simulink model "wholev5"  (R2018b)
settings: Solver=ode45  StartTime=0.0  StopTime=200  FixedStep=0.01  RelTol=1e-3
libraries: aerolibatmos2 x4
settings Model: Creator=hou2  LastModifiedBy=wq
settings DataIOCC: LimitDataPoints=on
settings OptimizationCC: DefaultParameterBehavior=Inlined  UseDivisionForNetSlopeComputation=on  UseFloatMulNetSlope=on  InlineInvariantSignals=on  PassReuseOutputArgsAs=Individual arguments  ZeroExternalMemoryAtStartup=off  ZeroInternalMemoryAtStartup=off  NoFixptDivByZeroProtection=on  EfficientFloat2IntCast=on  LifeSpan=1  OptimizeBlockOrder=speed  DifferentSizesBufferReuse=on
settings DebuggingCC: ParameterTunabilityLossMsg=error  AllowSymbolicDim=off  SFUnexpectedBacktrackingDiag=warning  SFNoUnconditionalDefaultTransitionDiag=warning  SFExecutionAtInitializationDiag=none
settings HardwareCC: ProdBitPerLong=64  ProdLongLongMode=on  ProdHWDeviceType=Intel->x86-64 (Linux 64)
settings ModelReferenceCC: PropagateSignalLabelsOutOfModel=off
settings SFSimCC: SimUseLocalCustomCode=off  MATLABDynamicMemAlloc=off
settings RTWCC: SystemTargetFile=ert.tlc  GenCodeOnly=on  TemplateMakefile=ert_default_tmf  GenerateReport=on  RTWUseLocalCustomCode=off  BuildConfiguration=Faster Runs  IncludeHyperlinkInReport=on  LaunchReport=on  TargetLang=C++  GenerateTraceInfo=on  GenerateTraceReport=on  GenerateTraceReportSl=on  GenerateTraceReportSf=on  GenerateTraceReportEml=on
settings CodeAppCC: ForceParamTrailComments=on  IgnoreCustomStorageClasses=off  OperatorAnnotations=on  SimulinkDataObjDesc=on  SFDataObjDesc=on  CustomSymbolStrGlobalVar=rt$N$M  CustomSymbolStrType=$N$M  CustomSymbolStrFcn=$N$M$F  CustomSymbolStrMacro=$N$M  InsertBlockDesc=on
settings ERTTargetCC: TargetLangStandard=C++03 (ISO)  GenerateSampleERTMain=on  IncludeMdlTerminateFcn=off  CombineSignalStateStructs=on  MultiInstanceERTCode=on  CodeInterfacePackaging=C++ class  SupportComplex=off  SupportContinuousTime=on  SupportNonInlinedSFcns=on  InlinedParameterPlacement=NonHierarchical  RootIOFormat=Structure reference  RTWCAPISignals=on  RTWCAPIParams=on  RTWCAPIStates=on  RTWCAPIRootIO=on  ERTCustomFileTemplate=example_file_process.tlc  ERTFilePackagingFormat=CompactWithDataFile
settings ConfigComp: CovMetricSettings=dw  CovHtmlReporting=on  CovSaveCumulativeToWorkspaceVar=on  CovSaveSingleToWorkspaceVar=on  CovExternalEMLEnable=off

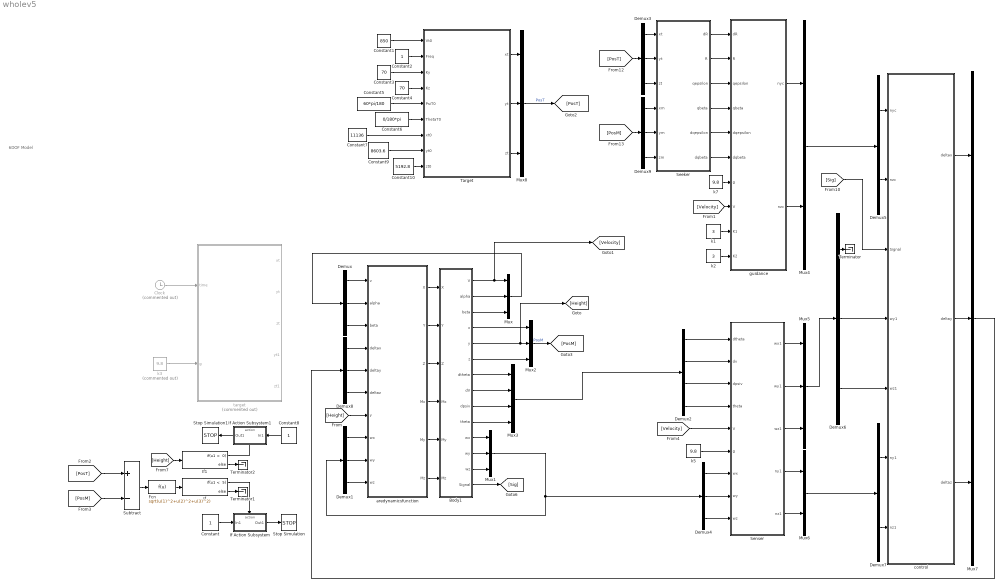
== system wholev5 ==
  note: 6DOF Model
  Body1 : Subsystem
  Clock : Clock  Commented=on
  Constant : Constant
  Constant1 : Constant  Value=850
  Constant10 : Constant  Value=5192.8
  Constant2 : Constant
  Constant3 : Constant  Value=70
  Constant4 : Constant  Value=70
  Constant5 : Constant  Value=60*pi/180
  Constant6 : Constant  Value=0/180*pi
  Constant7 : Constant  Value=11136
  Constant8 : Constant
  Constant9 : Constant  Value=8603.6
  Demux{,1,3..4,6,8..9} (7 alike) : Demux  Outputs=3
  Demux2 : Demux
  Demux5 : Demux  Outputs=2
  Demux7 : Demux  Outputs=2
  Fcn : Fcn  Expr=sqrt(u(1)^2+u(2)^2+u(3)^2)
  If : If  IfExpression="u1 <  5"
  If Action Subsystem : Subsystem  TreatAsAtomicUnit=on
  If Action Subsystem1 : Subsystem  TreatAsAtomicUnit=on
  If1 : If  IfExpression="u1 <  0"
  Mux{,1..2,5,7..8} (6 alike) : Mux  Inputs=3
  Mux3 : Mux
  Mux4 : Mux  Inputs=2
  Mux6 : Mux  Inputs=2
  Seeker : Subsystem
  Senser : Subsystem
  Stop Simulation : Stop
  Stop Simulation1 : Stop
  Subtract : Sum  Inputs=+-
  Target : Subsystem
  Terminator : Terminator
  Terminator1 : Terminator
  Terminator2 : Terminator
  aredynamicsfunction : Subsystem
  control : Subsystem
  guidance : Subsystem
  k1 : Constant  Value=3
  k2 : Constant  Value=3
  k3 : Constant  Commented=on  Value=9.8
  k5 : Constant  Value=9.8
  k7 : Constant  Value=9.8
  target : Subsystem  Commented=on
  wires:
  aredynamicsfunction/6(Mz) -> Body1/6(Mz)
  aredynamicsfunction/5(My) -> Body1/5(My)
  aredynamicsfunction/4(Mx) -> Body1/4(Mx)
  aredynamicsfunction/3(Z) -> Body1/3(Z)
  aredynamicsfunction/1(X) -> Body1/1(X)
  aredynamicsfunction/2(Y) -> Body1/2(Y)
  Seeker/3(qepsilon) -> guidance/3(qepsilon)
  Seeker/2(R) -> guidance/2(R)
  Seeker/6(dqbeta) -> guidance/6(dqbeta)
  Seeker/1(dR) -> guidance/1(dR)
  Seeker/4(qbeta) -> guidance/4(qbeta)
  Seeker/5(dqepsilon) -> guidance/5(dqepsilon)
  k1/1 -> guidance/9(K1)
  [Velocity] -> guidance/8(V)
  k2/1 -> guidance/10(K2)
  k7/1 -> guidance/7(g)
  Body1/1(V) -> Mux/1, [Velocity]
  Body1/2(alpha) -> Mux/2
  Body1/3(beta) -> Mux/3
  Mux/1 -> Demux/1
  Body1/11(wx) -> Mux1/1
  Body1/12(wy) -> Mux1/2
  Body1/13(wz) -> Mux1/3
  Mux1/1 -> Demux1/1, Demux4/1
  Body1/4(x) -> Mux2/1
  Body1/5(y) -> [Height], Mux2/2
  Body1/6(z) -> Mux2/3
  Mux2/1 -> [PosM]  "PosM"
  Body1/7(dtheta) -> Mux3/1
  Body1/8(dV) -> Mux3/2
  Body1/9(dpsiv) -> Mux3/3
  Body1/10(theta) -> Mux3/4
  [PosT] -> Subtract/1
  [PosM] -> Subtract/2
  Subtract/1 -> Fcn/1
  Fcn/1 -> If/1
  If/1 -> If Action Subsystem/Action
  If Action Subsystem/1(Out1) -> Stop Simulation/1
  If/2 -> Terminator1/1
  Constant/1 -> If Action Subsystem/1(In1)
  Demux2/1 -> Senser/1(dtheta)
  Demux2/2 -> Senser/2(dv)
  Demux2/3 -> Senser/3(dpsiv)
  Demux2/4 -> Senser/4(theta)
  [Velocity] -> Senser/5(V)
  k5/1 -> Senser/6(g)
  Demux4/1 -> Senser/7(wx)
  Demux4/2 -> Senser/8(wy)
  Demux4/3 -> Senser/9(wz)
  guidance/1(nyc) -> Mux4/1
  guidance/2(nzc) -> Mux4/2
  Senser/2(wy1) -> Mux5/2
  Senser/3(wz1) -> Mux5/3
  Senser/1("wx1 ") -> Mux5/1
  Senser/4(ny1) -> Mux6/1
  Senser/5(nz1) -> Mux6/2
  control/3(deltaz) -> Mux7/3
  control/2(deltay) -> Mux7/2
  control/1(deltax) -> Mux7/1
  Mux7/1 -> Demux8/1
  Demux/1 -> aredynamicsfunction/1(v)
  Demux/2 -> aredynamicsfunction/2(alpha)
  Demux/3 -> aredynamicsfunction/3(beta)
  Demux8/1 -> aredynamicsfunction/4(deltax)
  Demux8/2 -> aredynamicsfunction/5(deltay)
  Demux8/3 -> aredynamicsfunction/6(deltaz)
  Demux1/1 -> aredynamicsfunction/8(wx)
  Demux1/2 -> aredynamicsfunction/9(wy)
  Demux1/3 -> aredynamicsfunction/10(wz)
  [Height] -> aredynamicsfunction/7(y)
  Demux5/1 -> control/1(nyc)
  Demux5/2 -> control/2(nzc)
  Mux4/1 -> Demux5/1
  Demux6/2 -> control/4(wy1)
  Demux6/3 -> control/5(wz1)
  Mux5/1 -> Demux6/1
  Demux7/1 -> control/6(ny1)
  Demux7/2 -> control/7(nz1)
  Mux6/1 -> Demux7/1
  Constant1/1 -> Target/1(Vt0)
  Constant2/1 -> Target/2(Freq)
  Constant3/1 -> Target/3(Ky)
  Constant4/1 -> Target/4(Kz)
  Constant5/1 -> Target/5(PsiT0)
  Constant6/1 -> Target/6(ThetaT0)
  Clock/1 -> target/1(time)
  k3/1 -> target/2(g)
  Mux8/1 -> [PosT]  "PosT"
  [Height] -> If1/1
  If1/2 -> Terminator2/1
  If1/1 -> If Action Subsystem1/Action
  Constant8/1 -> If Action Subsystem1/1(In1)
  If Action Subsystem1/1(Out1) -> Stop Simulation1/1
  Target/1(xt) -> Mux8/1
  Target/2(yt) -> Mux8/2
  Target/3(zt) -> Mux8/3
  Mux3/1 -> Demux2/1
  Constant7/1 -> Target/7(xt0)
  Constant9/1 -> Target/8(yt0)
  Constant10/1 -> Target/9(zt0)
  Demux6/1 -> Terminator/1
  Body1/14(Signal) -> [Sig]
  [Sig] -> control/3(Signal)
  Demux3/1 -> Seeker/1(xt)
  Demux3/2 -> Seeker/2(yt)
  Demux3/3 -> Seeker/3(zt)
  Demux9/1 -> Seeker/4(xm)
  Demux9/3 -> Seeker/6(zm)
  Demux9/2 -> Seeker/5(ym)
  [PosT] -> Demux3/1
  [PosM] -> Demux9/1

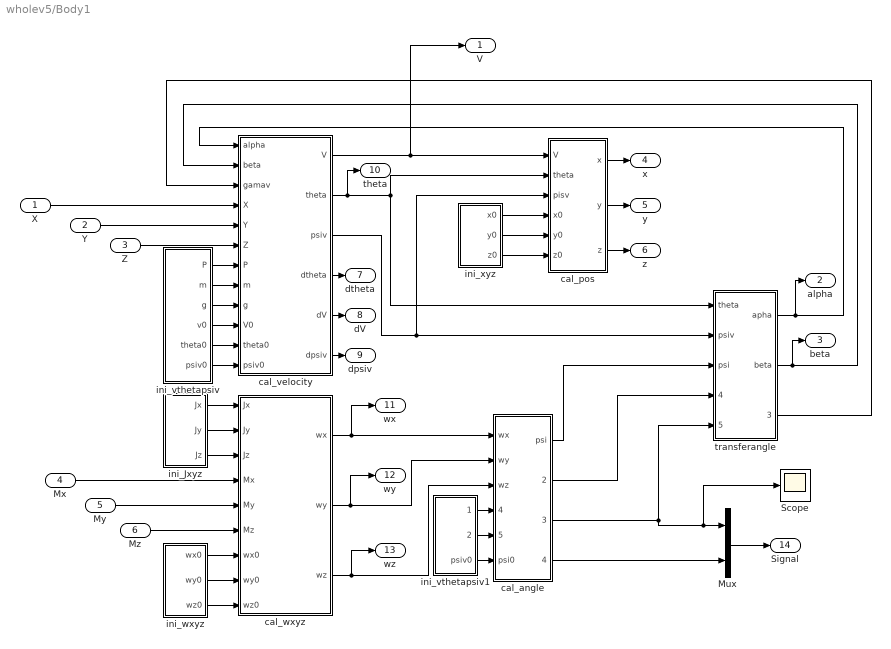
== system wholev5/Body1 ==
  X : Inport
  Y : Inport  Port=2
  Z : Inport  Port=3
  Mx : Inport  Port=4
  My : Inport  Port=5
  Mz : Inport  Port=6
  Mux : Mux  Inputs=2
  Scope : Scope
  cal_angle : Subsystem
  cal_pos : Subsystem
  cal_velocity : Subsystem
  cal_wxyz : Subsystem
  ini_Jxyz : Subsystem
  ini_vthetapsiv : Subsystem
  ini_vthetapsiv1 : Subsystem
  ini_wxyz : Subsystem
  ini_xyz : Subsystem
  transferangle : Subsystem
  V : Outport
  alpha : Outport  Port=2
  beta : Outport  Port=3
  x : Outport  Port=4
  y : Outport  Port=5
  z : Outport  Port=6
  dtheta : Outport  Port=7
  dV : Outport  Port=8
  dpsiv : Outport  Port=9
  theta : Outport  Port=10
  wx : Outport  Port=11
  wy : Outport  Port=12
  wz : Outport  Port=13
  Signal : Outport  Port=14
  wires:
  transferangle/3(gamav) -> cal_velocity/3(gamav)
  cal_velocity/2(theta) -> theta/1, transferangle/1(theta), cal_pos/2(theta)
  cal_velocity/3(psiv) -> cal_pos/3(pisv), transferangle/2(psiv)
  cal_velocity/1(V) -> cal_pos/1(V), V/1
  cal_wxyz/1(wx) -> cal_angle/1(wx), wx/1
  cal_wxyz/2(wy) -> cal_angle/2(wy), wy/1
  cal_wxyz/3(wz) -> cal_angle/3(wz), wz/1
  cal_angle/3(gama) -> Scope/1, Mux/1, transferangle/5(gama)
  cal_angle/2(Ctheta) -> transferangle/4(Ctheta)
  cal_angle/1(psi) -> transferangle/3(psi)
  transferangle/2(beta) -> beta/1, cal_velocity/2(beta)
  transferangle/1(apha) -> alpha/1, cal_velocity/1(alpha)
  cal_pos/1(x) -> x/1
  Y/1 -> cal_velocity/5(Y)
  Mx/1 -> cal_wxyz/4(Mx)
  Mz/1 -> cal_wxyz/6(Mz)
  Z/1 -> cal_velocity/6(Z)
  My/1 -> cal_wxyz/5(My)
  X/1 -> cal_velocity/4(X)
  ini_Jxyz/3(Jz) -> cal_wxyz/3(Jz)
  ini_Jxyz/2(Jy) -> cal_wxyz/2(Jy)
  ini_Jxyz/1(Jx) -> cal_wxyz/1(Jx)
  ini_vthetapsiv1/1(gama0) -> cal_angle/4(gama0)
  ini_wxyz/2(wy0) -> cal_wxyz/8(wy0)
  ini_wxyz/3(wz0) -> cal_wxyz/9(wz0)
  ini_wxyz/1(wx0) -> cal_wxyz/7(wx0)
  ini_xyz/1(x0) -> cal_pos/4(x0)
  ini_xyz/3(z0) -> cal_pos/6(z0)
  ini_xyz/2(y0) -> cal_pos/5(y0)
  cal_pos/2(y) -> y/1
  ini_vthetapsiv1/3(psiv0) -> cal_angle/6(psi0)
  ini_vthetapsiv1/2(Ctheta0) -> cal_angle/5(pha0)
  cal_pos/3(z) -> z/1
  cal_velocity/4(dtheta) -> dtheta/1
  cal_velocity/5(dV) -> dV/1
  cal_velocity/6(dpsiv) -> dpsiv/1
  ini_vthetapsiv/1(P) -> cal_velocity/7(P)
  ini_vthetapsiv/2(m) -> cal_velocity/8(m)
  ini_vthetapsiv/3(g) -> cal_velocity/9(g)
  ini_vthetapsiv/4(v0) -> cal_velocity/10(V0)
  ini_vthetapsiv/5(theta0) -> cal_velocity/11(theta0)
  ini_vthetapsiv/6(psiv0) -> cal_velocity/12(psiv0)
  cal_angle/4(Dgama) -> Mux/2
  Mux/1 -> Signal/1

== system wholev5/If Action Subsystem ==
  In1 : Inport
  Action Port : ActionPort  ActionType=then
  Out1 : Outport
  wires:
  In1/1 -> Out1/1

== system wholev5/If Action Subsystem1 ==
  In1 : Inport
  Action Port : ActionPort  ActionType=then
  Out1 : Outport
  wires:
  In1/1 -> Out1/1

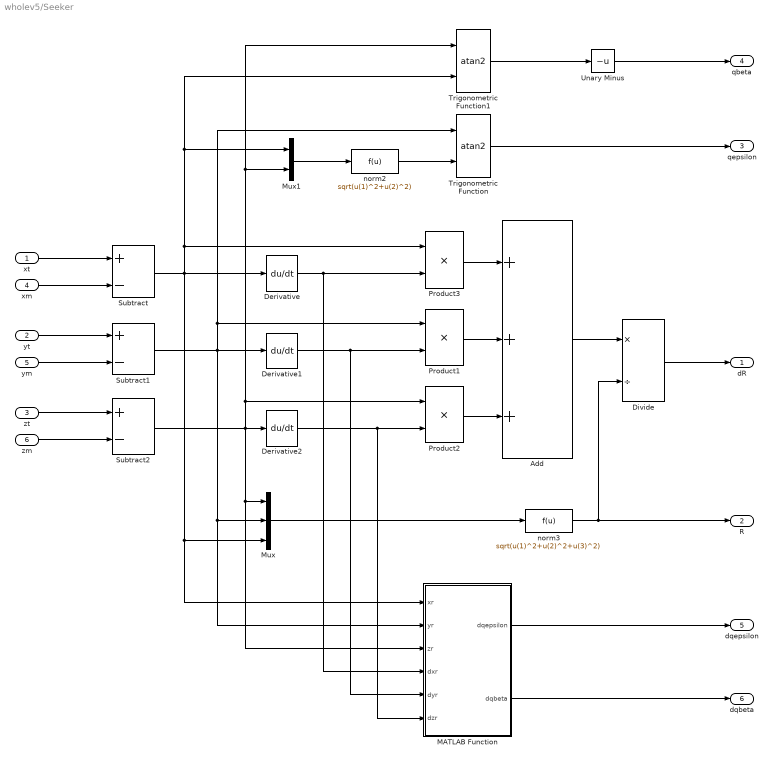
== system wholev5/Seeker ==
  xt : Inport
  yt : Inport  Port=2
  zt : Inport  Port=3
  xm : Inport  Port=4
  ym : Inport  Port=5
  zm : Inport  Port=6
  Add : Sum  Inputs=3
  Derivative : Derivative
  Derivative1 : Derivative
  Derivative2 : Derivative
  Divide : Product  Inputs=*/
  MATLAB Function : MATLAB Function  TreatAsAtomicUnit=on
  Mux : Mux  Inputs=3
  Mux1 : Mux  Inputs=2
  Product1 : Product
  Product2 : Product
  Product3 : Product
  Subtract : Sum  Inputs=+-
  Subtract1 : Sum  Inputs=+-
  Subtract2 : Sum  Inputs=+-
  Trigonometric Function : Trigonometry  Operator=atan2
  Trigonometric Function1 : Trigonometry  Operator=atan2
  Unary Minus : UnaryMinus
  norm2 : Fcn  Expr=sqrt(u(1)^2+u(2)^2)
  norm3 : Fcn  Expr=sqrt(u(1)^2+u(2)^2+u(3)^2)
  dR : Outport
  R : Outport  Port=2
  qepsilon : Outport  Port=3
  qbeta : Outport  Port=4
  dqepsilon : Outport  Port=5
  dqbeta : Outport  Port=6
  wires:
  Trigonometric Function/1 -> qepsilon/1
  Trigonometric Function1/1 -> Unary Minus/1
  Mux1/1 -> norm2/1
  Derivative/1 -> MATLAB Function/4(dxr), Product3/2
  Mux/1 -> norm3/1
  xm/1 -> Subtract/2
  Product3/1 -> Add/1
  zt/1 -> Subtract2/1
  Subtract1/1 -> MATLAB Function/2(yr), Mux/2, Derivative1/1, Trigonometric Function/1, Product1/1
  Subtract2/1 -> MATLAB Function/3(zr), Mux/1, Trigonometric Function1/1, Mux1/2, Product2/1, Derivative2/1
  Product1/1 -> Add/2
  Product2/1 -> Add/3
  Unary Minus/1 -> qbeta/1
  Divide/1 -> dR/1
  Add/1 -> Divide/1
  xt/1 -> Subtract/1
  ym/1 -> Subtract1/2
  Subtract/1 -> Mux/3, MATLAB Function/1(xr), Derivative/1, Trigonometric Function1/2, Mux1/1, Product3/1
  zm/1 -> Subtract2/2
  Derivative1/1 -> MATLAB Function/5(dyr), Product1/2
  yt/1 -> Subtract1/1
  norm2/1 -> Trigonometric Function/2
  norm3/1 -> R/1, Divide/2
  Derivative2/1 -> MATLAB Function/6(dzr), Product2/2
  MATLAB Function/2(dqbeta) -> dqbeta/1
  MATLAB Function/1(dqepsilon) -> dqepsilon/1

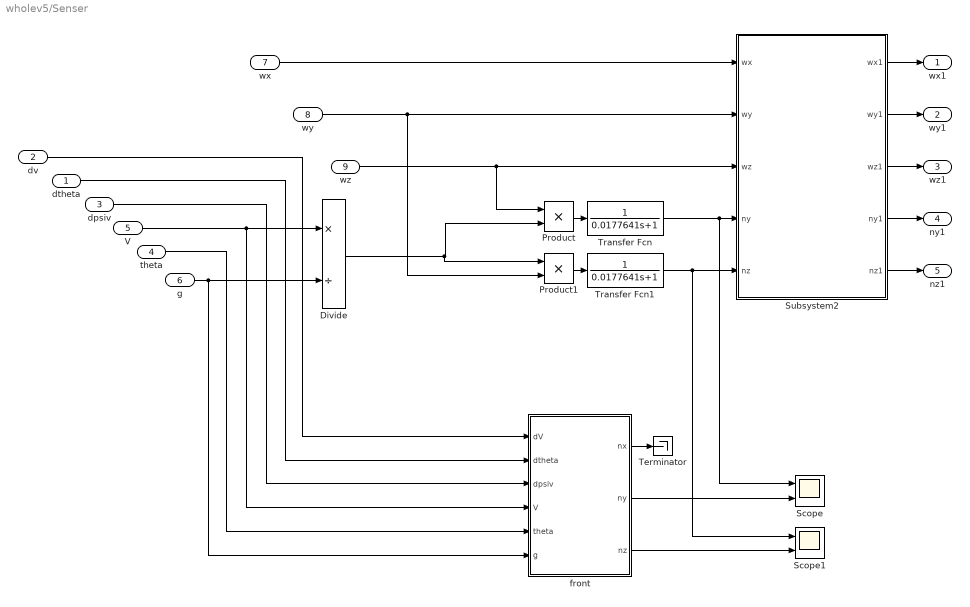
== system wholev5/Senser ==
  dtheta : Inport
  dv : Inport  Port=2
  dpsiv : Inport  Port=3
  theta : Inport  Port=4
  V : Inport  Port=5
  g : Inport  Port=6
  wx : Inport  Port=7
  wy : Inport  Port=8
  wz : Inport  Port=9
  Divide : Product  Inputs=*/
  Product : Product
  Product1 : Product
  Scope : Scope  NumInputPorts=2
  Scope1 : Scope  NumInputPorts=2
  Subsystem2 : Subsystem
  Terminator : Terminator
  Transfer Fcn : TransferFcn  Denominator=[0.0177641 1]
  Transfer Fcn1 : TransferFcn  Denominator=[0.0177641 1]
  front : Subsystem
  "wx1 " : Outport
  wy1 : Outport  Port=2
  wz1 : Outport  Port=3
  ny1 : Outport  Port=4
  nz1 : Outport  Port=5
  wires:
  wz/1 -> Product/1, Subsystem2/3(wz)
  dtheta/1 -> front/2(dtheta)
  wx/1 -> Subsystem2/1(wx)
  wy/1 -> Product1/2, Subsystem2/2(wy)
  dpsiv/1 -> front/3(dpsiv)
  theta/1 -> front/5(theta)
  dv/1 -> front/1(dV)
  Subsystem2/2(wy1) -> wy1/1
  V/1 -> front/4(V), Divide/1
  Subsystem2/1(wx1) -> "wx1 "/1
  Subsystem2/5(nz1) -> nz1/1
  g/1 -> front/6(g), Divide/2
  Subsystem2/3(wz1) -> wz1/1
  front/2(ny) -> Scope/2
  front/3(nz) -> Scope1/2
  Subsystem2/4(ny1) -> ny1/1
  front/1(nx) -> Terminator/1
  Transfer Fcn/1 -> Scope/1, Subsystem2/4(ny)
  Transfer Fcn1/1 -> Scope1/1, Subsystem2/5(nz)
  Product/1 -> Transfer Fcn/1
  Product1/1 -> Transfer Fcn1/1
  Divide/1 -> Product1/1, Product/2

== system wholev5/Target ==
  Vt0 : Inport
  Freq : Inport  Port=2
  Ky : Inport  Port=3
  Kz : Inport  Port=4
  PsiT0 : Inport  Port=5
  ThetaT0 : Inport  Port=6
  xt0 : Inport  Port=7
  yt0 : Inport  Port=8
  zt0 : Inport  Port=9
  Clock : Clock
  Integrator{,1..5} (6 alike) : Integrator  InitialConditionSource=external
  MATLAB Function : MATLAB Function  TreatAsAtomicUnit=on
  xt : Outport
  yt : Outport  Port=2
  zt : Outport  Port=3
  wires:
  zt0/1 -> Integrator2/2
  MATLAB Function/4(dx) -> Integrator4/1
  yt0/1 -> Integrator3/2
  Clock/1 -> MATLAB Function/4(t)
  Integrator1/1 -> MATLAB Function/3(Psi)
  MATLAB Function/2(dTheta) -> Integrator/1
  ThetaT0/1 -> Integrator/2
  PsiT0/1 -> Integrator1/2
  Freq/1 -> MATLAB Function/5(w)
  xt0/1 -> Integrator4/2
  Integrator3/1 -> yt/1
  Integrator4/1 -> xt/1
  Integrator/1 -> MATLAB Function/2(Theta)
  Kz/1 -> MATLAB Function/7(Kz)
  MATLAB Function/6(dz) -> Integrator2/1
  Integrator2/1 -> zt/1
  Ky/1 -> MATLAB Function/6(Ky)
  MATLAB Function/5(dy) -> Integrator3/1
  MATLAB Function/3(dPsi) -> Integrator1/1
  Vt0/1 -> Integrator5/2
  MATLAB Function/1(dV) -> Integrator5/1
  Integrator5/1 -> MATLAB Function/1(V)

== system wholev5/aredynamicsfunction ==
  v : Inport
  alpha : Inport  Port=2
  beta : Inport  Port=3
  deltax : Inport  Port=4
  deltay : Inport  Port=5
  deltaz : Inport  Port=6
  y : Inport  Port=7
  wx : Inport  Port=8
  wy : Inport  Port=9
  wz : Inport  Port=10
  Constant : Constant  Value=0
  cal_forceXYZ : Subsystem
  cal_momentMXZY : Subsystem
  X : Outport
  Y : Outport  Port=2
  Z : Outport  Port=3
  Mx : Outport  Port=4
  My : Outport  Port=5
  Mz : Outport  Port=6
  wires:
  Constant/1 -> cal_forceXYZ/3(Cx)
  v/1 -> cal_momentMXZY/2(V), cal_forceXYZ/2(V)
  cal_momentMXZY/1(Mx) -> Mx/1
  cal_forceXYZ/1(X) -> X/1
  cal_forceXYZ/2(Y) -> Y/1
  cal_momentMXZY/2(My) -> My/1
  cal_momentMXZY/3(Mz) -> Mz/1
  wz/1 -> cal_momentMXZY/10(wz)
  wx/1 -> cal_momentMXZY/8(wx)
  cal_forceXYZ/3(Z) -> Z/1
  deltaz/1 -> cal_momentMXZY/7(deltaz), cal_forceXYZ/7(deltaz)
  beta/1 -> cal_forceXYZ/5(beta), cal_momentMXZY/4(beta)
  deltay/1 -> cal_momentMXZY/6(deltay), cal_forceXYZ/6(deltay)
  alpha/1 -> cal_momentMXZY/3(alpha), cal_forceXYZ/4(alpha)
  y/1 -> cal_forceXYZ/1(y), cal_momentMXZY/1(y)
  wy/1 -> cal_momentMXZY/9(wy)
  deltax/1 -> cal_momentMXZY/5(deltax)

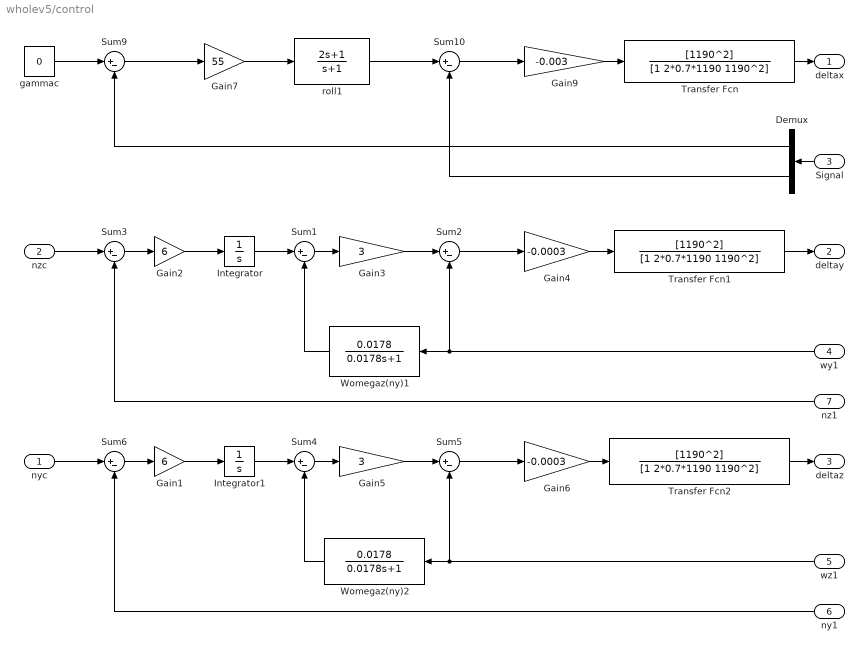
== system wholev5/control ==
  nyc : Inport
  nzc : Inport  Port=2
  Signal : Inport  Port=3
  wy1 : Inport  Port=4
  wz1 : Inport  Port=5
  ny1 : Inport  Port=6
  nz1 : Inport  Port=7
  " Womegaz(ny)1" : TransferFcn  Numerator=[0.0178]  Denominator=[0.0178 1]
  " Womegaz(ny)2" : TransferFcn  Numerator=[0.0178]  Denominator=[0.0178 1]
  Demux : Demux  Outputs=2
  Gain1 : Gain  Gain=6
  Gain2 : Gain  Gain=6
  Gain3 : Gain  Gain=3
  Gain4 : Gain  Gain=-0.0003
  Gain5 : Gain  Gain=3
  Gain6 : Gain  Gain=-0.0003
  Gain7 : Gain  Gain=55
  Gain9 : Gain  Gain=-0.003
  Integrator : Integrator
  Integrator1 : Integrator
  Sum{1..6,9..10} (8 alike) : Sum  Inputs=|+-
  Transfer Fcn : TransferFcn  Numerator=[1190^2]  Denominator=[1 2*0.7*1190 1190^2]
  Transfer Fcn1 : TransferFcn  Numerator=[1190^2]  Denominator=[1 2*0.7*1190 1190^2]
  Transfer Fcn2 : TransferFcn  Numerator=[1190^2]  Denominator=[1 2*0.7*1190 1190^2]
  gammac : Constant  Value=0
  roll1 : TransferFcn  Numerator=[2 1]  Denominator=[1 1]
  deltax : Outport
  deltay : Outport  Port=2
  deltaz : Outport  Port=3
  wires:
  Transfer Fcn/1 -> deltax/1
  Transfer Fcn1/1 -> deltay/1
  Transfer Fcn2/1 -> deltaz/1
  Gain2/1 -> Integrator/1
  Integrator/1 -> Sum1/1
  Sum2/1 -> Gain4/1
  Gain3/1 -> Sum2/1
  Sum1/1 -> Gain3/1
  Sum3/1 -> Gain2/1
  nzc/1 -> Sum3/1
  nz1/1 -> Sum3/2
  " Womegaz(ny)1"/1 -> Sum1/2
  wy1/1 -> Sum2/2, " Womegaz(ny)1"/1
  Gain4/1 -> Transfer Fcn1/1
  Gain1/1 -> Integrator1/1
  Integrator1/1 -> Sum4/1
  Sum5/1 -> Gain6/1
  Gain5/1 -> Sum5/1
  Sum4/1 -> Gain5/1
  Sum6/1 -> Gain1/1
  nyc/1 -> Sum6/1
  ny1/1 -> Sum6/2
  " Womegaz(ny)2"/1 -> Sum4/2
  wz1/1 -> Sum5/2, " Womegaz(ny)2"/1
  Gain6/1 -> Transfer Fcn2/1
  Signal/1 -> Demux/1
  Gain7/1 -> roll1/1
  Demux/1 -> Sum9/2
  roll1/1 -> Sum10/1
  Sum9/1 -> Gain7/1
  Sum10/1 -> Gain9/1
  gammac/1 -> Sum9/1
  Demux/2 -> Sum10/2
  Gain9/1 -> Transfer Fcn/1

== system wholev5/guidance ==
  dR : Inport
  R : Inport  Port=2
  qepsilon : Inport  Port=3
  qbeta : Inport  Port=4
  dqepsilon : Inport  Port=5
  dqbeta : Inport  Port=6
  g : Inport  Port=7
  V : Inport  Port=8
  K1 : Inport  Port=9
  K2 : Inport  Port=10
  Divide : Product  Inputs=/*
  Product : Product  Inputs=3
  Product1 : Product  Inputs=3
  Terminator{,1..3} (4 alike) : Terminator
  nyc : Outport
  nzc : Outport  Port=2
  wires:
  R/1 -> Terminator1/1
  qepsilon/1 -> Terminator2/1
  g/1 -> Divide/1
  dR/1 -> Terminator/1
  V/1 -> Divide/2
  qbeta/1 -> Terminator3/1
  Product1/1 -> nzc/1
  dqbeta/1 -> Product1/3
  dqepsilon/1 -> Product/1
  K2/1 -> Product1/2
  K1/1 -> Product/2
  Divide/1 -> Product1/1, Product/3
  Product/1 -> nyc/1

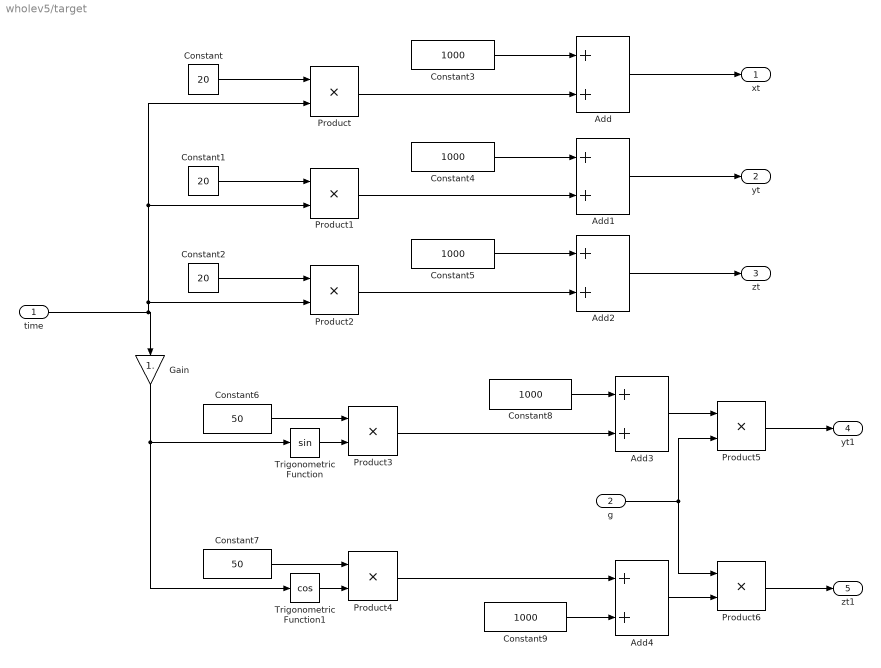
== system wholev5/target ==
  time : Inport
  g : Inport  Port=2
  Add{,1..4} (5 alike) : Sum
  Constant : Constant  Value=20
  Constant1 : Constant  Value=20
  Constant2 : Constant  Value=20
  Constant{3..5,8..9} (5 alike) : Constant  Value=1000
  Constant6 : Constant  Value=50
  Constant7 : Constant  Value=50
  Gain : Gain  Gain=1.
  Product{,1..6} (7 alike) : Product
  Trigonometric Function : Trigonometry
  Trigonometric Function1 : Trigonometry  Operator=cos
  xt : Outport
  yt : Outport  Port=2
  zt : Outport  Port=3
  yt1 : Outport  Port=4
  zt1 : Outport  Port=5
  wires:
  Product6/1 -> zt1/1
  Trigonometric Function/1 -> Product3/2
  Constant7/1 -> Product4/1
  Constant3/1 -> Add/1
  Constant5/1 -> Add2/1
  Constant/1 -> Product/1
  Product2/1 -> Add2/2
  Constant4/1 -> Add1/1
  Product1/1 -> Add1/2
  g/1 -> Product6/1, Product5/2
  Trigonometric Function1/1 -> Product4/2
  Constant6/1 -> Product3/1
  Add2/1 -> zt/1
  Constant1/1 -> Product1/1
  Product5/1 -> yt1/1
  Product/1 -> Add/2
  Constant2/1 -> Product2/1
  Add1/1 -> yt/1
  time/1 -> Gain/1, Product/2, Product1/2, Product2/2
  Add/1 -> xt/1
  Gain/1 -> Trigonometric Function/1, Trigonometric Function1/1
  Constant8/1 -> Add3/1
  Product3/1 -> Add3/2
  Add3/1 -> Product5/1
  Constant9/1 -> Add4/2
  Product4/1 -> Add4/1
  Add4/1 -> Product6/2

== system wholev5/Body1/cal_angle ==
  wx : Inport
  wy : Inport  Port=2
  wz : Inport  Port=3
  gama0 : Inport  Port=4
  pha0 : Inport  Port=5
  psi0 : Inport  Port=6
  Divide : Product  Inputs=**
  Divide1 : Product  Inputs=**
  Divide2 : Product  Inputs=/*
  Integrator : Integrator  InitialConditionSource=external
  Subtract : Sum  Inputs=+-
  Trigonometric Function : Trigonometry  Operator=cos
  Trigonometric Function1 : Trigonometry
  Trigonometric Function2 : Trigonometry  Operator=cos
  cal_Ctheta : Subsystem
  psi : Outport
  Ctheta : Outport  Port=2
  gama : Outport  Port=3
  Dgama : Outport  Port=4
  wires:
  Trigonometric Function/1 -> Divide/1
  wy/1 -> cal_Ctheta/2(wy), Divide/2
  wz/1 -> cal_Ctheta/4(wz), Divide1/2
  cal_Ctheta/2(gama) -> Trigonometric Function1/1, Trigonometric Function/1, gama/1
  Divide/1 -> Subtract/1
  psi0/1 -> Integrator/2
  Integrator/1 -> psi/1
  Trigonometric Function1/1 -> Divide1/1
  Trigonometric Function2/1 -> Divide2/1
  wx/1 -> cal_Ctheta/1(wx)
  Subtract/1 -> Divide2/2
  Divide1/1 -> Subtract/2
  cal_Ctheta/1(Ctheta) -> Trigonometric Function2/1, Ctheta/1
  pha0/1 -> cal_Ctheta/5(pha0)
  Divide2/1 -> Integrator/1
  gama0/1 -> cal_Ctheta/3(gama0)
  cal_Ctheta/3(Dgama) -> Dgama/1

== system wholev5/Body1/cal_pos ==
  note: x坐标的初始值
  note: z坐标的初始值
  V : Inport
  theta : Inport  Port=2
  pisv : Inport  Port=3
  x0 : Inport  Port=4
  y0 : Inport  Port=5
  z0 : Inport  Port=6
  Gain2 : Gain  Gain=-1
  Integrator : Integrator  InitialConditionSource=external
  Integrator1 : Integrator  InitialConditionSource=external
  Integrator2 : Integrator  InitialConditionSource=external
  Product : Product  Inputs=3
  Product1 : Product
  Product2 : Product  Inputs=3
  Trigonometric Function : Trigonometry  Operator=cos
  Trigonometric Function1 : Trigonometry  Operator=cos
  Trigonometric Function2 : Trigonometry
  Trigonometric Function3 : Trigonometry
  x : Outport
  y : Outport  Port=2
  z : Outport  Port=3
  wires:
  Integrator/1 -> x/1
  theta/1 -> Trigonometric Function2/1, Trigonometric Function/1
  pisv/1 -> Trigonometric Function3/1, Trigonometric Function1/1
  Trigonometric Function1/1 -> Product/2
  Trigonometric Function/1 -> Product2/3, Product/1
  x0/1 -> Integrator/2
  Product/1 -> Integrator/1
  V/1 -> Gain2/1, Product/3, Product1/1
  Trigonometric Function2/1 -> Product1/2
  Product1/1 -> Integrator1/1
  Integrator1/1 -> y/1
  y0/1 -> Integrator1/2
  Product2/1 -> Integrator2/1
  z0/1 -> Integrator2/2
  Trigonometric Function3/1 -> Product2/2
  Gain2/1 -> Product2/1
  Integrator2/1 -> z/1

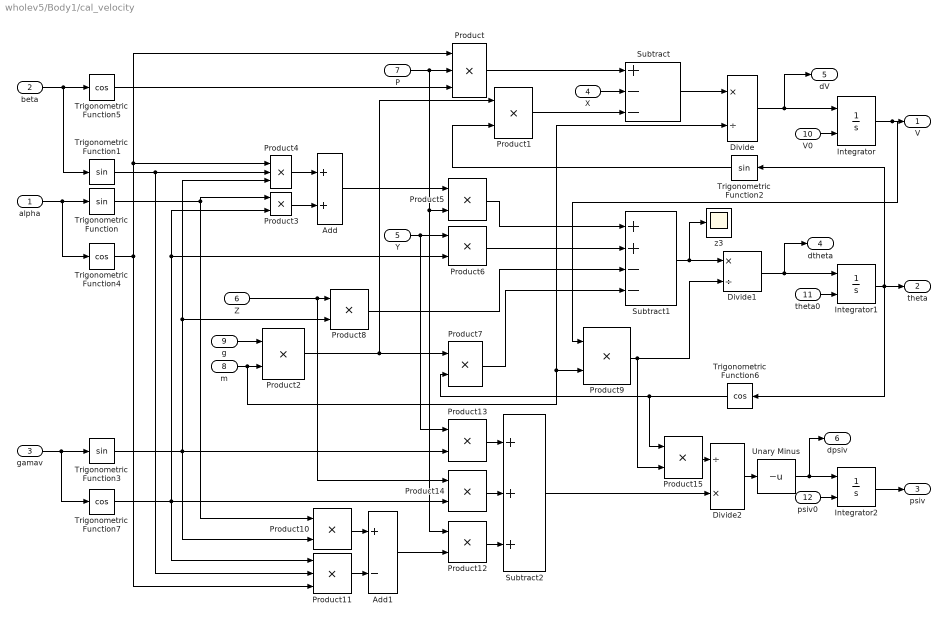
== system wholev5/Body1/cal_velocity ==
  alpha : Inport
  beta : Inport  Port=2
  gamav : Inport  Port=3
  X : Inport  Port=4
  Y : Inport  Port=5
  Z : Inport  Port=6
  P : Inport  Port=7
  m : Inport  Port=8
  g : Inport  Port=9
  V0 : Inport  Port=10
  theta0 : Inport  Port=11
  psiv0 : Inport  Port=12
  Add : Sum
  Add1 : Sum  Inputs=+-
  Divide : Product  Inputs=*/
  Divide1 : Product  Inputs=*/
  Divide2 : Product  Inputs=/*
  Integrator : Integrator  InitialConditionSource=external
  Integrator1 : Integrator  InitialConditionSource=external
  Integrator2 : Integrator  InitialConditionSource=external
  Product : Product  Inputs=3
  Product{1..3,5..10,12..15} (13 alike) : Product
  Product11 : Product  Inputs=3
  Product4 : Product  Inputs=3
  Subtract : Sum  Inputs=+--
  Subtract1 : Sum  Inputs=++--
  Subtract2 : Sum  Inputs=+++
  Trigonometric Function{,1..3} (4 alike) : Trigonometry
  Trigonometric Function{4..7} (4 alike) : Trigonometry  Operator=cos
  Unary Minus : UnaryMinus
  z3 : Scope
  V : Outport
  theta : Outport  Port=2
  psiv : Outport  Port=3
  dtheta : Outport  Port=4
  dV : Outport  Port=5
  dpsiv : Outport  Port=6
  wires:
  Trigonometric Function2/1 -> Product1/2
  Trigonometric Function7/1 -> Product11/1, Product6/2, Product3/2, Product14/2
  X/1 -> Subtract/2
  Trigonometric Function1/1 -> Product11/2, Product4/2
  Product1/1 -> Subtract/3
  Product3/1 -> Add/2
  Product4/1 -> Add/1
  Trigonometric Function4/1 -> Product11/3, Product/1, Product4/1
  Product/1 -> Subtract/1
  alpha/1 -> Trigonometric Function/1, Trigonometric Function4/1
  beta/1 -> Trigonometric Function1/1, Trigonometric Function5/1
  g/1 -> Product2/1
  Product2/1 -> Product7/1, Product1/1
  Trigonometric Function/1 -> Product3/1, Product10/1
  m/1 -> Product2/2, Product9/2, Divide/2
  Trigonometric Function5/1 -> Product/3
  gamav/1 -> Trigonometric Function3/1, Trigonometric Function7/1
  P/1 -> Product12/1, Product5/2, Product/2
  Trigonometric Function3/1 -> Product8/2, Product4/3, Product10/2, Product13/2
  Subtract/1 -> Divide/1
  Integrator1/1 -> theta/1, Trigonometric Function6/1, Trigonometric Function2/1
  Y/1 -> Product13/1, Product6/1
  Product10/1 -> Add1/1
  Subtract2/1 -> Divide2/2
  Subtract1/1 -> z3/1, Divide1/1
  Product11/1 -> Add1/2
  Product13/1 -> Subtract2/1
  Trigonometric Function6/1 -> Product7/2, Product15/1
  Divide2/1 -> Unary Minus/1
  Product14/1 -> Subtract2/2
  Product6/1 -> Subtract1/2
  Product9/1 -> Divide1/2, Product15/2
  Product5/1 -> Subtract1/1
  Add1/1 -> Product12/2
  Product8/1 -> Subtract1/3
  Z/1 -> Product8/1, Product14/1
  Add/1 -> Product5/1
  Product15/1 -> Divide2/1
  Product12/1 -> Subtract2/3
  Product7/1 -> Subtract1/4
  Unary Minus/1 -> dpsiv/1, Integrator2/1
  V0/1 -> Integrator/2
  psiv0/1 -> Integrator2/2
  Divide1/1 -> dtheta/1, Integrator1/1
  Integrator2/1 -> psiv/1
  theta0/1 -> Integrator1/2
  Integrator/1 -> Product9/1, V/1
  Divide/1 -> Integrator/1, dV/1

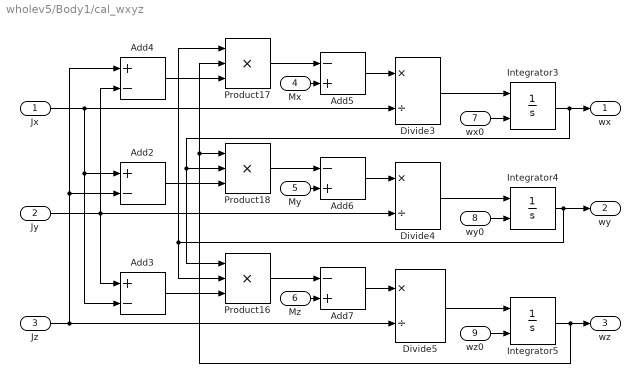
== system wholev5/Body1/cal_wxyz ==
  Jx : Inport
  Jy : Inport  Port=2
  Jz : Inport  Port=3
  Mx : Inport  Port=4
  My : Inport  Port=5
  Mz : Inport  Port=6
  wx0 : Inport  Port=7
  wy0 : Inport  Port=8
  wz0 : Inport  Port=9
  Add2 : Sum  Inputs=+-
  Add3 : Sum  Inputs=+-
  Add4 : Sum  Inputs=+-
  Add5 : Sum  Inputs=-+
  Add6 : Sum  Inputs=-+
  Add7 : Sum  Inputs=-+
  Divide3 : Product  Inputs=*/
  Divide4 : Product  Inputs=*/
  Divide5 : Product  Inputs=*/
  Integrator3 : Integrator  InitialConditionSource=external
  Integrator4 : Integrator  InitialConditionSource=external
  Integrator5 : Integrator  InitialConditionSource=external
  Product16 : Product  Inputs=3
  Product17 : Product  Inputs=3
  Product18 : Product  Inputs=3
  wx : Outport
  wy : Outport  Port=2
  wz : Outport  Port=3
  wires:
  Integrator4/1 -> wy/1, Product16/2, Product17/1
  Jx/1 -> Add3/2, Add2/1, Divide3/2
  Jy/1 -> Add3/1, Add4/2, Divide4/2
  Jz/1 -> Add4/1, Add2/2, Divide5/2
  wx0/1 -> Integrator3/2
  Integrator5/1 -> wz/1, Product17/2, Product18/1
  Divide4/1 -> Integrator4/1
  wz0/1 -> Integrator5/2
  Product17/1 -> Add5/1
  wy0/1 -> Integrator4/2
  Add7/1 -> Divide5/1
  Add3/1 -> Product16/3
  My/1 -> Add6/2
  Divide3/1 -> Integrator3/1
  Divide5/1 -> Integrator5/1
  Add5/1 -> Divide3/1
  Product18/1 -> Add6/1
  Product16/1 -> Add7/1
  Mx/1 -> Add5/2
  Integrator3/1 -> wx/1, Product16/1, Product18/2
  Add4/1 -> Product17/3
  Add2/1 -> Product18/3
  Mz/1 -> Add7/2
  Add6/1 -> Divide4/1

== system wholev5/Body1/ini_Jxyz ==
  b : Constant  Value=0.0071
  b0 : Constant  Value=0.1863
  b1 : Constant  Value=0.1863
  Jx : Outport
  Jy : Outport  Port=2
  Jz : Outport  Port=3
  wires:
  b1/1 -> Jz/1
  b0/1 -> Jy/1
  b/1 -> Jx/1

== system wholev5/Body1/ini_vthetapsiv ==
  Gain : Gain  Gain=pi/180
  Gain1 : Gain  Gain=pi/180
  b : Constant  Value=1000
  b0 : Constant  Value=45
  b1 : Constant  Value=0
  b2 : Constant  Value=0
  b3 : Constant  Value=4.9718
  b4 : Constant  Value=9.8
  P : Outport
  m : Outport  Port=2
  g : Outport  Port=3
  v0 : Outport  Port=4
  theta0 : Outport  Port=5
  psiv0 : Outport  Port=6
  wires:
  b1/1 -> Gain1/1
  b0/1 -> Gain/1
  b/1 -> v0/1
  b4/1 -> g/1
  b3/1 -> m/1
  b2/1 -> P/1
  Gain/1 -> theta0/1
  Gain1/1 -> psiv0/1

== system wholev5/Body1/ini_vthetapsiv1 ==
  Gain : Gain  Gain=pi/180
  b : Constant  Value=0
  b0 : Constant  Value=45
  b1 : Constant  Value=0
  gama0 : Outport
  Ctheta0 : Outport  Port=2
  psiv0 : Outport  Port=3
  wires:
  b/1 -> gama0/1
  b0/1 -> Gain/1
  b1/1 -> psiv0/1
  Gain/1 -> Ctheta0/1

== system wholev5/Body1/ini_wxyz ==
  b : Constant  Value=0
  b0 : Constant  Value=0
  b1 : Constant  Value=0
  wx0 : Outport
  wy0 : Outport  Port=2
  wz0 : Outport  Port=3
  wires:
  b/1 -> wx0/1
  b0/1 -> wy0/1
  b1/1 -> wz0/1

== system wholev5/Body1/ini_xyz ==
  b : Constant  Value=0
  b0 : Constant  Value=0
  b1 : Constant  Value=0
  x0 : Outport
  y0 : Outport  Port=2
  z0 : Outport  Port=3
  wires:
  b1/1 -> z0/1
  b0/1 -> y0/1
  b/1 -> x0/1

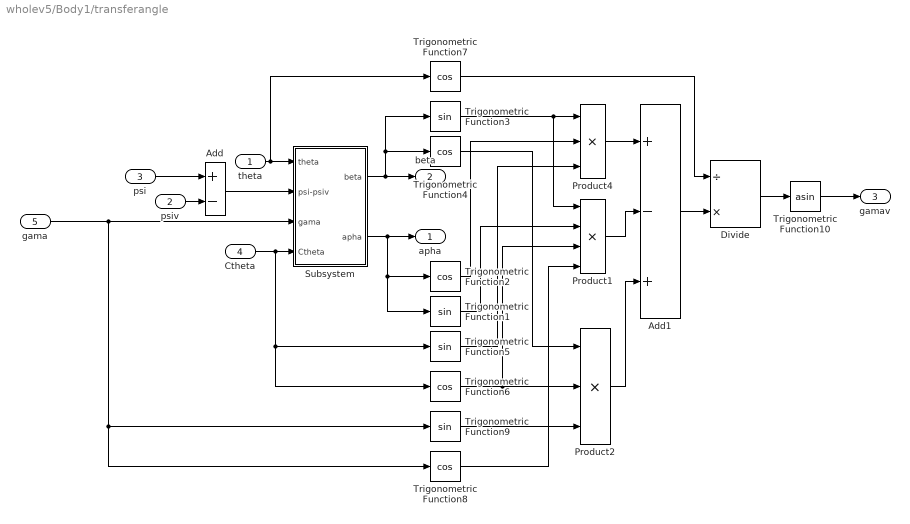
== system wholev5/Body1/transferangle ==
  theta : Inport
  psiv : Inport  Port=2
  psi : Inport  Port=3
  Ctheta : Inport  Port=4
  gama : Inport  Port=5
  Add : Sum  Inputs=+-
  Add1 : Sum  Inputs=+-+
  Divide : Product  Inputs=/*
  Product1 : Product  Inputs=4
  Product2 : Product  Inputs=3
  Product4 : Product  Inputs=3
  Subsystem : Subsystem
  Trigonometric Function{1,3,5,9} (4 alike) : Trigonometry
  Trigonometric Function10 : Trigonometry  Operator=asin
  Trigonometric Function{2,4,6..8} (5 alike) : Trigonometry  Operator=cos
  apha : Outport
  beta : Outport  Port=2
  gamav : Outport  Port=3
  wires:
  Trigonometric Function2/1 -> Product4/2
  Trigonometric Function1/1 -> Product1/2
  Trigonometric Function3/1 -> Product1/1, Product4/1
  Product1/1 -> Add1/2
  Trigonometric Function6/1 -> Product2/2, Product1/3
  Trigonometric Function4/1 -> Product2/1
  Product4/1 -> Add1/1
  Trigonometric Function7/1 -> Divide/1
  Product2/1 -> Add1/3
  Trigonometric Function8/1 -> Product1/4
  Add1/1 -> Divide/2
  Ctheta/1 -> Trigonometric Function6/1, Trigonometric Function5/1, Subsystem/4(Ctheta)
  theta/1 -> Subsystem/1(theta), Trigonometric Function7/1
  gama/1 -> Trigonometric Function8/1, Trigonometric Function9/1, Subsystem/3(gama)
  Subsystem/2(apha) -> apha/1, Trigonometric Function1/1, Trigonometric Function2/1
  Add/1 -> Subsystem/2(psi-psiv)
  Subsystem/1(beta) -> beta/1, Trigonometric Function3/1, Trigonometric Function4/1
  Trigonometric Function9/1 -> Product2/3
  Trigonometric Function5/1 -> Product4/3
  psiv/1 -> Add/2
  psi/1 -> Add/1
  Divide/1 -> Trigonometric Function10/1
  Trigonometric Function10/1 -> gamav/1

== system wholev5/Senser/Subsystem2 ==
  wx : Inport
  wy : Inport  Port=2
  wz : Inport  Port=3
  ny : Inport  Port=4
  nz : Inport  Port=5
  Accel1 : TransferFcn  Denominator=[0.00003481 0.00708 1 ]
  Accel2 : TransferFcn  Denominator=[0.00003481 0.00708 1 ]
  Accel3 : TransferFcn  Denominator=[0.00003481 0.00708 1 ]
  Geroscope1 : TransferFcn  Denominator=[0.000036 0.0084 1 ]
  Geroscope2 : TransferFcn  Denominator=[0.000036 0.0084 1 ]
  wx1 : Outport
  wy1 : Outport  Port=2
  wz1 : Outport  Port=3
  ny1 : Outport  Port=4
  nz1 : Outport  Port=5
  wires:
  nz/1 -> Geroscope2/1
  ny/1 -> Geroscope1/1
  Geroscope2/1 -> nz1/1
  Geroscope1/1 -> ny1/1
  wz/1 -> Accel3/1
  wy/1 -> Accel2/1
  wx/1 -> Accel1/1
  Accel1/1 -> wx1/1
  Accel2/1 -> wy1/1
  Accel3/1 -> wz1/1

== system wholev5/Senser/front ==
  dV : Inport
  dtheta : Inport  Port=2
  dpsiv : Inport  Port=3
  V : Inport  Port=4
  theta : Inport  Port=5
  g : Inport  Port=6
  Add : Sum
  Add1 : Sum
  Constant : Constant
  Divide : Product  Inputs=*/
  Product : Product
  Product1 : Product
  Product2 : Product
  Product3 : Product  Inputs=3
  Trigonometric Function : Trigonometry
  Trigonometric Function1 : Trigonometry  Operator=cos
  Unary Minus : UnaryMinus
  nx : Outport
  ny : Outport  Port=2
  nz : Outport  Port=3
  wires:
  V/1 -> Product/1
  dpsiv/1 -> Product3/3
  Trigonometric Function1/1 -> Add1/2, Product3/2
  Add/1 -> nx/1
  Trigonometric Function/1 -> Add/2
  Add1/1 -> ny/1
  Unary Minus/1 -> Product3/1
  Product/1 -> Product2/2, Unary Minus/1
  Constant/1 -> Divide/1
  theta/1 -> Trigonometric Function1/1, Trigonometric Function/1
  Product3/1 -> nz/1
  g/1 -> Divide/2
  Product1/1 -> Add/1
  dV/1 -> Product1/2
  dtheta/1 -> Product2/1
  Product2/1 -> Add1/1
  Divide/1 -> Product/2, Product1/1

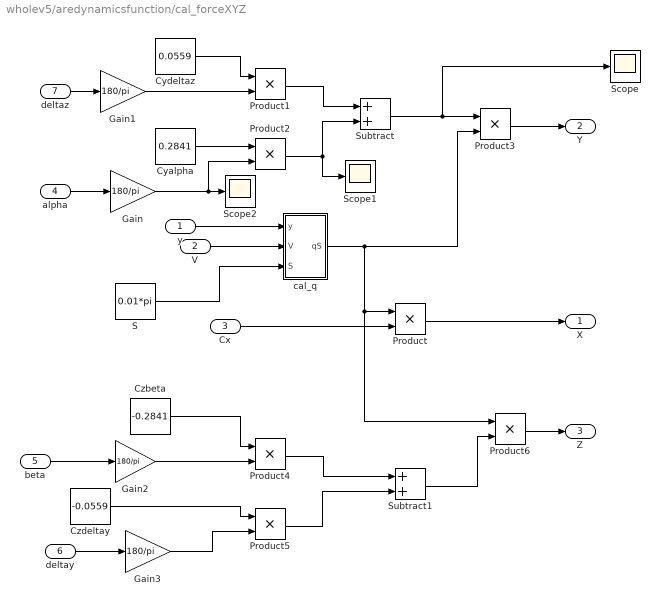
== system wholev5/aredynamicsfunction/cal_forceXYZ ==
  y : Inport
  V : Inport  Port=2
  Cx : Inport  Port=3
  alpha : Inport  Port=4
  beta : Inport  Port=5
  deltay : Inport  Port=6
  deltaz : Inport  Port=7
  Cyalpha : Constant  Value=0.2841
  Cydeltaz : Constant  Value=0.0559
  Czbeta : Constant  Value=-0.2841
  Czdeltay : Constant  Value=-0.0559
  Gain{,1..3} (4 alike) : Gain  Gain=180/pi
  Product{,1..6} (7 alike) : Product
  S : Constant  Value=0.01*pi
  Scope : Scope
  Scope1 : Scope
  Scope2 : Scope
  Subtract : Sum
  Subtract1 : Sum
  cal_q : Subsystem
  X : Outport
  Y : Outport  Port=2
  Z : Outport  Port=3
  wires:
  Cx/1 -> Product/2
  Cyalpha/1 -> Product2/1
  Product2/1 -> Scope1/1, Subtract/2
  Product1/1 -> Subtract/1
  Product3/1 -> Y/1
  Cydeltaz/1 -> Product1/1
  cal_q/1(qS) -> Product3/2, Product6/1, Product/1
  Subtract/1 -> Scope/1, Product3/1
  Product/1 -> X/1
  S/1 -> cal_q/3(S)
  y/1 -> cal_q/1(y)
  V/1 -> cal_q/2(V)
  Czdeltay/1 -> Product5/1
  Product4/1 -> Subtract1/1
  Product5/1 -> Subtract1/2
  Czbeta/1 -> Product4/1
  Subtract1/1 -> Product6/2
  Product6/1 -> Z/1
  alpha/1 -> Gain/1
  Gain/1 -> Scope2/1, Product2/2
  deltaz/1 -> Gain1/1
  Gain1/1 -> Product1/2
  Gain2/1 -> Product4/2
  beta/1 -> Gain2/1
  deltay/1 -> Gain3/1
  Gain3/1 -> Product5/2

== system wholev5/aredynamicsfunction/cal_momentMXZY ==
  y : Inport
  V : Inport  Port=2
  alpha : Inport  Port=3
  beta : Inport  Port=4
  deltax : Inport  Port=5
  deltay : Inport  Port=6
  deltaz : Inport  Port=7
  wx : Inport  Port=8
  wy : Inport  Port=9
  wz : Inport  Port=10
  cal_momentMX : Subsystem
  cal_momentMY : Subsystem
  cal_momentMZ : Subsystem
  Mx : Outport
  My : Outport  Port=2
  Mz : Outport  Port=3
  wires:
  V/1 -> cal_momentMY/2(V), cal_momentMX/2(V), cal_momentMZ/2(V)
  deltaz/1 -> cal_momentMZ/3(deltaz)
  deltax/1 -> cal_momentMX/3(deltax)
  cal_momentMY/1(My) -> My/1
  wz/1 -> cal_momentMZ/4(wz)
  deltay/1 -> cal_momentMY/3(deltay)
  cal_momentMZ/1(Mz) -> Mz/1
  wx/1 -> cal_momentMX/4(wx)
  cal_momentMX/1(Mx) -> Mx/1
  alpha/1 -> cal_momentMX/5(alpha), cal_momentMZ/5(alpha)
  wy/1 -> cal_momentMY/4(wy)
  beta/1 -> cal_momentMY/5(beta)
  y/1 -> cal_momentMZ/1(y), cal_momentMY/1(y), cal_momentMX/1(y)

== system wholev5/Body1/cal_angle/cal_Ctheta ==
  wx : Inport
  wy : Inport  Port=2
  gama0 : Inport  Port=3
  wz : Inport  Port=4
  pha0 : Inport  Port=5
  Integrator : Integrator  InitialConditionSource=external
  Product : Product
  Product1 : Product
  Subtract : Sum
  Trigonometric Function : Trigonometry
  Trigonometric Function1 : Trigonometry  Operator=cos
  cal_r : Subsystem
  Ctheta : Outport
  gama : Outport  Port=2
  Dgama : Outport  Port=3
  wires:
  pha0/1 -> Integrator/2
  Integrator/1 -> cal_r/2(Ctheta), Ctheta/1
  wx/1 -> cal_r/1(wx)
  gama0/1 -> cal_r/4(gama0)
  Product/1 -> Subtract/1
  Product1/1 -> Subtract/2
  Trigonometric Function1/1 -> Product1/1
  Subtract/1 -> Integrator/1
  cal_r/1(gama) -> gama/1, Trigonometric Function/1, Trigonometric Function1/1
  wy/1 -> Product/1, cal_r/3(wy)
  wz/1 -> cal_r/5(wz), Product1/2
  Trigonometric Function/1 -> Product/2
  cal_r/2(Dgama) -> Dgama/1

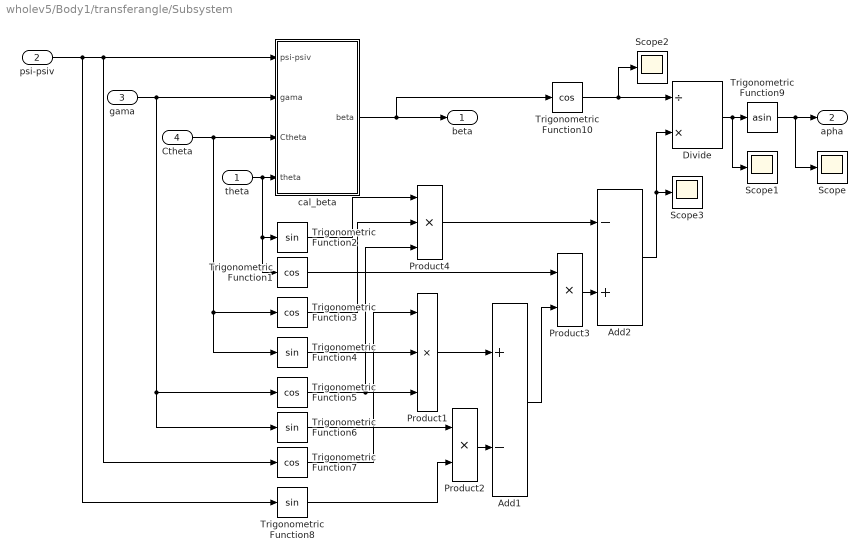
== system wholev5/Body1/transferangle/Subsystem ==
  theta : Inport
  psi-psiv : Inport  Port=2
  gama : Inport  Port=3
  Ctheta : Inport  Port=4
  Add1 : Sum  Inputs=+-
  Add2 : Sum  Inputs=-+
  Divide : Product  Inputs=/*
  Product1 : Product  Inputs=3
  Product2 : Product
  Product3 : Product
  Product4 : Product  Inputs=3
  Scope{,1..3} (4 alike) : Scope
  Trigonometric Function{1,3,5,7,10} (5 alike) : Trigonometry  Operator=cos
  Trigonometric Function{2,4,6,8} (4 alike) : Trigonometry
  Trigonometric Function9 : Trigonometry  Operator=asin
  cal_beta : Subsystem
  beta : Outport
  apha : Outport  Port=2
  wires:
  cal_beta/1(beta) -> Trigonometric Function10/1, beta/1
  Ctheta/1 -> Trigonometric Function4/1, Trigonometric Function3/1, cal_beta/3(Ctheta)
  gama/1 -> cal_beta/2(gama), Trigonometric Function6/1, Trigonometric Function5/1
  theta/1 -> Trigonometric Function1/1, Trigonometric Function2/1, cal_beta/4(theta)
  Trigonometric Function4/1 -> Product1/2
  Product3/1 -> Add2/2
  Product2/1 -> Add1/2
  Trigonometric Function2/1 -> Product4/1
  Add1/1 -> Product3/2
  Product4/1 -> Add2/1
  Trigonometric Function5/1 -> Product4/3, Product1/3
  Trigonometric Function3/1 -> Product4/2
  Trigonometric Function6/1 -> Product2/1
  Trigonometric Function8/1 -> Product2/2
  Trigonometric Function7/1 -> Product1/1
  Trigonometric Function1/1 -> Product3/1
  Product1/1 -> Add1/1
  Trigonometric Function9/1 -> Scope/1, apha/1
  Add2/1 -> Scope3/1, Divide/2
  psi-psiv/1 -> cal_beta/1(psi-psiv), Trigonometric Function7/1, Trigonometric Function8/1
  Trigonometric Function10/1 -> Scope2/1, Divide/1
  Divide/1 -> Scope1/1, Trigonometric Function9/1

== system wholev5/aredynamicsfunction/cal_forceXYZ/cal_q ==
  y : Inport
  V : Inport  Port=2
  S : Inport  Port=3
  COESA Atmosphere Model : aerolibatmos2/COESA Atmosphere Model  units=Metric (MKS)  spec=1976 COESA-extended U.S. Standard Atmosphere  model=Profile  profile_var=High temperature  profile_percent=1%  profile_alt=5 km (16404 ft)  envelope_var=High temperature  envelope_percent=1%  action=Warning
  Constant : Constant  Value=0.5
  Divide : Product  Inputs=**
  Divide1 : Product  Inputs=4
  Mux : Mux  Inputs=3
  Terminator : Terminator
  z : Scope
  qS : Outport
  wires:
  y/1 -> COESA Atmosphere Model/1
  COESA Atmosphere Model/4 -> Divide1/4, z/1
  S/1 -> Divide/2
  Divide1/1 -> Divide/1
  V/1 -> Divide1/2, Divide1/3
  Divide/1 -> qS/1
  Constant/1 -> Divide1/1
  COESA Atmosphere Model/1 -> Mux/1
  COESA Atmosphere Model/2 -> Mux/2
  COESA Atmosphere Model/3 -> Mux/3
  Mux/1 -> Terminator/1

== system wholev5/aredynamicsfunction/cal_momentMXZY/cal_momentMX ==
  y : Inport
  V : Inport  Port=2
  deltax : Inport  Port=3
  wx : Inport  Port=4
  alpha : Inport  Port=5
  Gain : Gain  Gain=180/pi
  Gain1 : Gain  Gain=180/pi
  Gain2 : Gain  Gain=180/pi
  L : Constant
  MATLAB Function1 : MATLAB Function  TreatAsAtomicUnit=on
  Product : Product
  Product1 : Product
  Product2 : Product  Inputs=3
  S : Constant  Value=0.01*pi
  Subsystem1 : Subsystem
  Subtract : Sum
  cal_q : Subsystem
  mxdeltax : Constant  Value=-0.0062
  Mx : Outport
  wires:
  Product2/1 -> Mx/1
  Product1/1 -> Subtract/2
  L/1 -> Product2/3
  Subsystem1/1(res) -> Product/2
  V/1 -> cal_q/2(V), Subsystem1/2(v)
  S/1 -> cal_q/3(S)
  Subtract/1 -> Product2/1
  y/1 -> cal_q/1(y)
  Product/1 -> Subtract/1
  mxdeltax/1 -> Product1/2
  wx/1 -> Gain/1
  deltax/1 -> Gain1/1
  Gain1/1 -> Product1/1
  cal_q/1(qS) -> Product2/2
  Gain/1 -> Subsystem1/1(In1)
  alpha/1 -> Gain2/1
  Gain2/1 -> MATLAB Function1/1(alpha)
  MATLAB Function1/1(mxwx) -> Product/1

== system wholev5/aredynamicsfunction/cal_momentMXZY/cal_momentMY ==
  y : Inport
  V : Inport  Port=2
  deltay : Inport  Port=3
  wy : Inport  Port=4
  beta : Inport  Port=5
  Gain : Gain  Gain=180/pi
  Gain1 : Gain  Gain=180/pi
  Gain2 : Gain  Gain=180/pi
  L : Constant
  Product : Product
  Product1 : Product
  Product2 : Product  Inputs=3
  Product3 : Product
  S : Constant  Value=0.01*pi
  Subsystem : Subsystem
  Subtract : Sum  Inputs=+++
  cal_q : Subsystem
  mybeta : Constant  Value=-0.0104
  mydelaty : Constant  Value=-0.0206
  mywy : Constant  Value=-0.0026
  My : Outport
  wires:
  Product2/1 -> My/1
  cal_q/1(qS) -> Product2/2
  L/1 -> Product2/3
  mywy/1 -> Product/2
  V/1 -> cal_q/2(V), Subsystem/2(v)
  S/1 -> cal_q/3(S)
  Subtract/1 -> Product2/1
  y/1 -> cal_q/1(y)
  mydelaty/1 -> Product1/2
  mybeta/1 -> Product3/1
  Product1/1 -> Subtract/3
  Product/1 -> Subtract/2
  Product3/1 -> Subtract/1
  Gain/1 -> Product3/2
  beta/1 -> Gain/1
  wy/1 -> Gain1/1
  deltay/1 -> Gain2/1
  Gain2/1 -> Product1/1
  Gain1/1 -> Subsystem/1(In1)
  Subsystem/1(res) -> Product/1

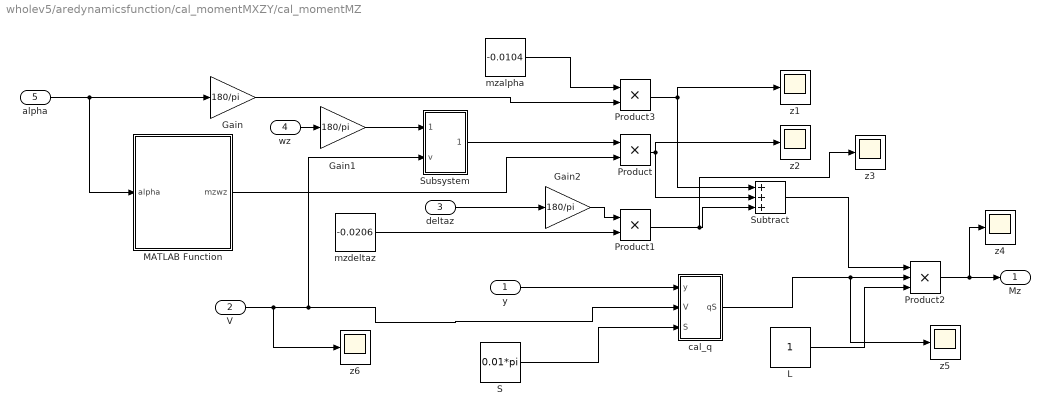
== system wholev5/aredynamicsfunction/cal_momentMXZY/cal_momentMZ ==
  y : Inport
  V : Inport  Port=2
  deltaz : Inport  Port=3
  wz : Inport  Port=4
  alpha : Inport  Port=5
  Gain : Gain  Gain=180/pi
  Gain1 : Gain  Gain=180/pi
  Gain2 : Gain  Gain=180/pi
  L : Constant
  MATLAB Function : MATLAB Function  TreatAsAtomicUnit=on
  Product : Product
  Product1 : Product
  Product2 : Product  Inputs=3
  Product3 : Product
  S : Constant  Value=0.01*pi
  Subsystem : Subsystem
  Subtract : Sum  Inputs=+++
  cal_q : Subsystem
  mzalpha : Constant  Value=-0.0104
  mzdeltaz : Constant  Value=-0.0206
  z{1..6} (6 alike) : Scope
  Mz : Outport
  wires:
  Product2/1 -> z4/1, Mz/1
  L/1 -> Product2/3
  MATLAB Function/1(mzwz) -> Product/2
  V/1 -> z6/1, cal_q/2(V), Subsystem/2(v)
  S/1 -> cal_q/3(S)
  Subtract/1 -> Product2/1
  y/1 -> cal_q/1(y)
  mzdeltaz/1 -> Product1/2
  mzalpha/1 -> Product3/1
  Product1/1 -> z3/1, Subtract/3
  Product/1 -> Subtract/2, z2/1
  Product3/1 -> Subtract/1, z1/1
  alpha/1 -> MATLAB Function/1(alpha), Gain/1
  Gain/1 -> Product3/2
  wz/1 -> Gain1/1
  deltaz/1 -> Gain2/1
  Gain2/1 -> Product1/1
  cal_q/1(qS) -> z5/1, Product2/2
  Gain1/1 -> Subsystem/1(In1)
  Subsystem/1(res) -> Product/1

== system wholev5/Body1/cal_angle/cal_Ctheta/cal_r ==
  wx : Inport
  Ctheta : Inport  Port=2
  wy : Inport  Port=3
  gama0 : Inport  Port=4
  wz : Inport  Port=5
  Divide1 : Product  Inputs=**
  Divide2 : Product  Inputs=**
  Divide3 : Product  Inputs=**
  Integrator : Integrator  InitialConditionSource=external
  Subtract : Sum  Inputs=+-
  Subtract1 : Sum  Inputs=+-
  Trigonometric Function : Trigonometry  Operator=tan
  Trigonometric Function1 : Trigonometry  Operator=cos
  Trigonometric Function2 : Trigonometry
  gama : Outport
  Dgama : Outport  Port=2
  wires:
  wx/1 -> Subtract/1
  Trigonometric Function/1 -> Divide1/1
  Ctheta/1 -> Trigonometric Function/1
  Subtract/1 -> Dgama/1, Integrator/1
  gama0/1 -> Integrator/2
  Integrator/1 -> gama/1, Trigonometric Function2/1, Trigonometric Function1/1
  Trigonometric Function1/1 -> Divide2/1
  wy/1 -> Divide2/2
  Divide2/1 -> Subtract1/1
  Trigonometric Function2/1 -> Divide3/1
  wz/1 -> Divide3/2
  Divide3/1 -> Subtract1/2
  Subtract1/1 -> Divide1/2
  Divide1/1 -> Subtract/2

== system wholev5/Body1/transferangle/Subsystem/cal_beta ==
  psi-psiv : Inport
  gama : Inport  Port=2
  Ctheta : Inport  Port=3
  theta : Inport  Port=4
  Add1 : Sum  Inputs=+-
  Add2 : Sum
  Product : Product
  Product1 : Product  Inputs=3
  Product2 : Product
  Product3 : Product  Inputs=3
  Trigonometric Function{,1..2,6} (4 alike) : Trigonometry  Operator=cos
  Trigonometric Function{3..5,7} (4 alike) : Trigonometry
  Trigonometric Function8 : Trigonometry  Operator=asin
  beta : Outport
  wires:
  theta/1 -> Trigonometric Function7/1, Trigonometric Function1/1
  gama/1 -> Trigonometric Function5/1, Trigonometric Function/1
  psi-psiv/1 -> Trigonometric Function2/1, Trigonometric Function3/1
  Trigonometric Function/1 -> Product/1
  Trigonometric Function3/1 -> Product/2
  Ctheta/1 -> Trigonometric Function6/1, Trigonometric Function4/1
  Trigonometric Function2/1 -> Product1/2
  Trigonometric Function4/1 -> Product1/3
  Trigonometric Function5/1 -> Product1/1, Product3/2
  Trigonometric Function6/1 -> Product3/3
  Trigonometric Function7/1 -> Product3/1
  Product2/1 -> Add1/1
  Product3/1 -> Add1/2
  Add1/1 -> Trigonometric Function8/1
  Trigonometric Function8/1 -> beta/1
  Product1/1 -> Add2/2
  Product/1 -> Add2/1
  Trigonometric Function1/1 -> Product2/2
  Add2/1 -> Product2/1

== system wholev5/aredynamicsfunction/cal_momentMXZY/cal_momentMX/Subsystem1 ==
  In1 : Inport
  v : Inport  Port=2
  Constant : Constant  Value=2
  Divide : Product  Inputs=*//
  res : Outport
  wires:
  In1/1 -> Divide/1
  Constant/1 -> Divide/3
  Divide/1 -> res/1
  v/1 -> Divide/2

== system wholev5/aredynamicsfunction/cal_momentMXZY/cal_momentMX/cal_q ==
  y : Inport
  V : Inport  Port=2
  S : Inport  Port=3
  COESA Atmosphere Model : aerolibatmos2/COESA Atmosphere Model  units=Metric (MKS)  spec=1976 COESA-extended U.S. Standard Atmosphere  model=Profile  profile_var=High temperature  profile_percent=1%  profile_alt=5 km (16404 ft)  envelope_var=High temperature  envelope_percent=1%  action=Warning
  Constant : Constant  Value=0.5
  Divide : Product  Inputs=**
  Divide1 : Product  Inputs=4
  Mux : Mux  Inputs=3
  Terminator : Terminator
  z : Scope
  qS : Outport
  wires:
  y/1 -> COESA Atmosphere Model/1
  COESA Atmosphere Model/4 -> Divide1/4, z/1
  S/1 -> Divide/2
  Divide1/1 -> Divide/1
  V/1 -> Divide1/2, Divide1/3
  Divide/1 -> qS/1
  Constant/1 -> Divide1/1
  COESA Atmosphere Model/1 -> Mux/1
  COESA Atmosphere Model/2 -> Mux/2
  COESA Atmosphere Model/3 -> Mux/3
  Mux/1 -> Terminator/1

== system wholev5/aredynamicsfunction/cal_momentMXZY/cal_momentMY/Subsystem ==
  In1 : Inport
  v : Inport  Port=2
  Constant : Constant  Value=2
  Divide : Product  Inputs=*//
  res : Outport
  wires:
  In1/1 -> Divide/1
  Constant/1 -> Divide/3
  Divide/1 -> res/1
  v/1 -> Divide/2

== system wholev5/aredynamicsfunction/cal_momentMXZY/cal_momentMY/cal_q ==
  y : Inport
  V : Inport  Port=2
  S : Inport  Port=3
  COESA Atmosphere Model : aerolibatmos2/COESA Atmosphere Model  units=Metric (MKS)  spec=1976 COESA-extended U.S. Standard Atmosphere  model=Profile  profile_var=High temperature  profile_percent=1%  profile_alt=5 km (16404 ft)  envelope_var=High temperature  envelope_percent=1%  action=Warning
  Constant : Constant  Value=0.5
  Divide : Product  Inputs=**
  Divide1 : Product  Inputs=4
  Mux : Mux  Inputs=3
  Terminator : Terminator
  z : Scope
  qS : Outport
  wires:
  y/1 -> COESA Atmosphere Model/1
  COESA Atmosphere Model/4 -> Divide1/4, z/1
  S/1 -> Divide/2
  Divide1/1 -> Divide/1
  V/1 -> Divide1/2, Divide1/3
  Divide/1 -> qS/1
  Constant/1 -> Divide1/1
  COESA Atmosphere Model/1 -> Mux/1
  COESA Atmosphere Model/2 -> Mux/2
  COESA Atmosphere Model/3 -> Mux/3
  Mux/1 -> Terminator/1

== system wholev5/aredynamicsfunction/cal_momentMXZY/cal_momentMZ/Subsystem ==
  In1 : Inport
  v : Inport  Port=2
  Constant : Constant  Value=2
  Divide : Product  Inputs=*//
  res : Outport
  wires:
  In1/1 -> Divide/1
  Constant/1 -> Divide/3
  Divide/1 -> res/1
  v/1 -> Divide/2

== system wholev5/aredynamicsfunction/cal_momentMXZY/cal_momentMZ/cal_q ==
  y : Inport
  V : Inport  Port=2
  S : Inport  Port=3
  COESA Atmosphere Model : aerolibatmos2/COESA Atmosphere Model  units=Metric (MKS)  spec=1976 COESA-extended U.S. Standard Atmosphere  model=Profile  profile_var=High temperature  profile_percent=1%  profile_alt=5 km (16404 ft)  envelope_var=High temperature  envelope_percent=1%  action=Warning
  Constant : Constant  Value=0.5
  Divide : Product  Inputs=**
  Divide1 : Product  Inputs=4
  Mux : Mux  Inputs=3
  Terminator : Terminator
  z : Scope
  qS : Outport
  wires:
  y/1 -> COESA Atmosphere Model/1
  COESA Atmosphere Model/4 -> Divide1/4, z/1
  S/1 -> Divide/2
  Divide1/1 -> Divide/1
  V/1 -> Divide1/2, Divide1/3
  Divide/1 -> qS/1
  Constant/1 -> Divide1/1
  COESA Atmosphere Model/1 -> Mux/1
  COESA Atmosphere Model/2 -> Mux/2
  COESA Atmosphere Model/3 -> Mux/3
  Mux/1 -> Terminator/1

== matlab function wholev5/Target/MATLAB Function ==
  data: V input; dV output; Theta input; dTheta output; Psi input; t input; w input; Ky input; Kz input; dPsi output; dx output; dy output; dz output
function [dV,dTheta,dPsi,dx,dy,dz] = target(V,Theta,Psi,t,w,Ky,Kz)
    dV = -9.81*sin(Theta);
    dTheta = (Ky * sin(w*t)-9.81*cos(Theta)) / V;
    dPsi = - Kz * cos(w*t) / V / cos(Theta);
    dx = V * cos(Theta) * cos(Psi);
    dy = V * sin(Theta);
    dz = - V * cos(Theta) * sin(Psi);
end

== matlab function wholev5/aredynamicsfunction/cal_momentMXZY/cal_momentMX/MATLAB Function1 ==
  data: alpha input; mxwx output
function mxwx  = fcn(alpha)
alpha1=[-6 -4 -2 0 2 4 6];
mxwx1=[-0.0082 -0.0078 -0.0078 -0.0074 -0.0078 -0.0078 -0.0082];
mxwx=interp1(alpha1,mxwx1,alpha,'linear','extrap');

== matlab function wholev5/aredynamicsfunction/cal_momentMXZY/cal_momentMZ/MATLAB Function ==
  data: alpha input; mzwz output
function mzwz  = fcn(alpha)
alpha1=[-6 -4 -2 0 2 4 6];
mzwz1=[-0.0097 -0.015 -0.0191 -0.0236 -0.0296 -0.0351 -0.0413];
mzwz=interp1(alpha1,mzwz1,alpha,'linear','extrap');

== matlab function wholev5/Seeker/MATLAB Function ==
  data: xr input; dqepsilon output; yr input; zr input; dxr input; dyr input; dzr input; dqbeta output
function [dqepsilon,dqbeta] = fcn(xr,yr,zr,dxr,dyr,dzr)
dqepsilon=( (xr^2+zr^2) * dyr - yr * (xr*dxr+zr*dzr) ) / ...
          ( (xr^2+yr^2+zr^2) * sqrt(xr^2+zr^2) );
dqbeta=( zr*dxr - xr*dzr ) / ...
       ( xr^2 + zr^2 );
